simulink model "rigid_body_dynamics"  (R2024b)
settings: Solver=VariableStepAuto  StartTime=0.0  StopTime=10.0  RelTol=1e-3
libraries: robotmaniplib x3
settings Model: Creator=spenu  LastModifiedBy=spenu

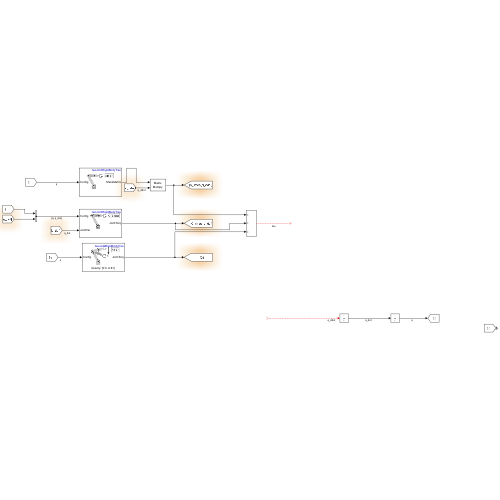
[thumbnail: Simulink's stored preview of the top-level diagram]
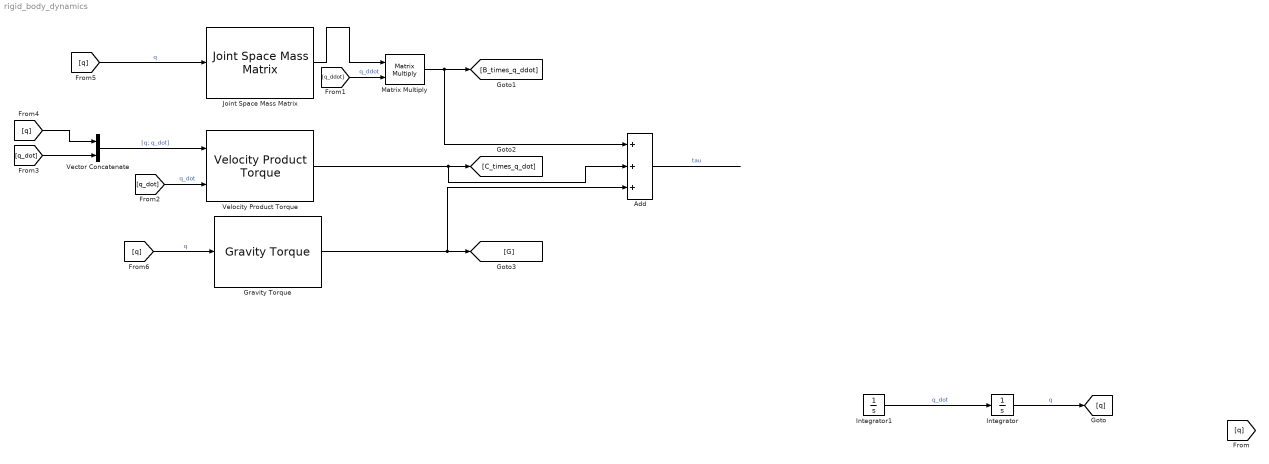
== system rigid_body_dynamics ==
  Add : Sum  Inputs=+++
  Gravity Torque : robotmaniplib/Gravity Torque  RigidBodyTree=twoJointRigidBodyTree  SimulateUsing=Interpreted execution
  Integrator : Integrator
  Integrator1 : Integrator
  Joint Space Mass Matrix : robotmaniplib/Joint Space Mass Matrix  RigidBodyTree=twoJointRigidBodyTree  SimulateUsing=Interpreted execution
  Matrix Multiply : Product  Multiplication=Matrix(*)
  Vector Concatenate : Concatenate
  Velocity Product Torque : robotmaniplib/Velocity Product Torque  RigidBodyTree=twoJointRigidBodyTree  SimulateUsing=Interpreted execution
  wires:
  Integrator/1 -> [q]  "q"
  Integrator1/1 -> Integrator/1  "q_dot"
  ? -> Integrator1/1  "q_ddot"
  Joint Space Mass Matrix/1 -> Matrix Multiply/1
  [q] -> Joint Space Mass Matrix/1  "q"
  [q_ddot] -> Matrix Multiply/2  "q_ddot"
  [q_dot] -> Velocity Product Torque/2  "q_dot"
  Vector Concatenate/1 -> Velocity Product Torque/1  "[q; q_dot]"
  [q_dot] -> Vector Concatenate/2
  [q] -> Vector Concatenate/1
  [q] -> Gravity Torque/1  "q"
  Add/1 -> ?  "tau"
  Velocity Product Torque/1 -> Add/2, [C_times_q_dot]
  Gravity Torque/1 -> Add/3, [G]
  Matrix Multiply/1 -> Add/1, [B_times_q_ddot]
